simulink model "communicationExcavatorCANOldShit"  (R2025a)
settings: Solver=VariableStepAuto  StartTime=0.0  StopTime=Inf  RelTol=1e-3
undefined symbols (not defined in the file or in its folder): canChannel, SampleTime
libraries: canlib x10, canmsglib x8, simulink_extras x4, simulink x3, aerolibanimutils x1, sl3dlib x1
settings Model: Creator=Viktor Traktor  LastModifiedBy=Viktor Traktor
settings SolverCC: DecoupledContinuousIntegration=on

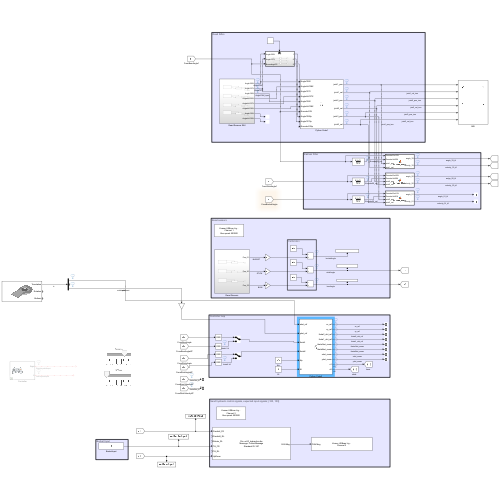
[thumbnail: Simulink's stored preview of the top-level diagram]
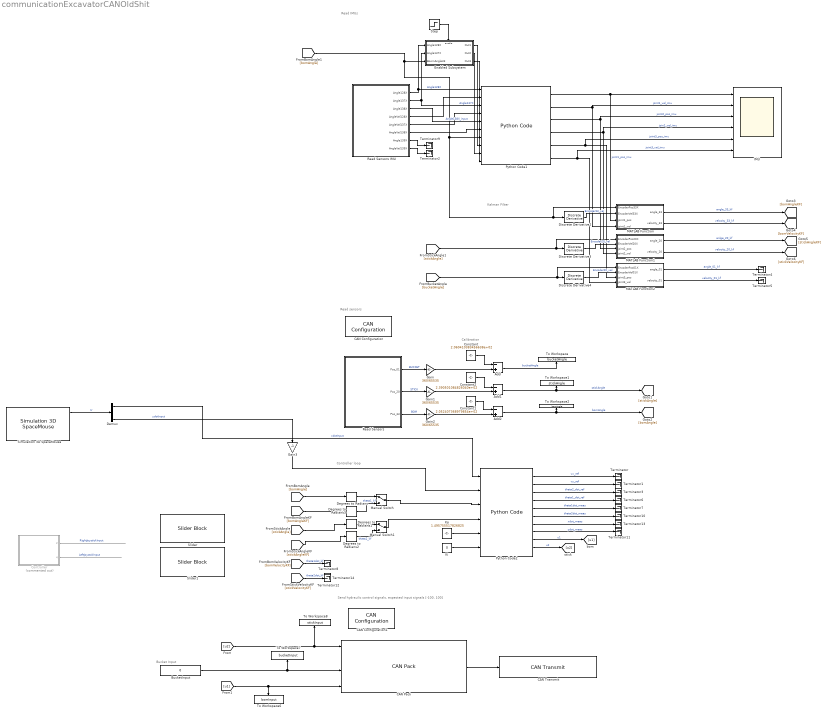
== system communicationExcavatorCANOldShit ==
  note: Controller loop
  note: Read sensors
  note: Send hydraulic control signals, expected input signals [-100, 100]
  note: Calibration
  note: Bucket Input
  note: Kalman Filter
  note: Read IMUs
  Add : Sum  Inputs=-+
  Add1 : Sum  Inputs=-+
  Add2 : Sum  Inputs=-+
  BucketInput : Constant  Value=0
  CAN Configuration : canlib/CAN Configuration  BlockHandle=6751.0004  Device=Kvaser USBcan Light 1 (Channel 1)  DeviceMenu=Kvaser USBcan Light 1 (Channel 1)  ObjConstructor=canChannel('Kvaser', 'USBcan Light 1', 1)  BusSpeed=500000  EnableBitParameters=off  SJW=1  TSEG1=4  TSEG2=3  NSamples=1  AckMode=Normal
  CAN Configuration1 : canlib/CAN Configuration  BlockHandle=6752.0004  Device=Kvaser USBcan Light 1 (Channel 2)  DeviceMenu=Kvaser USBcan Light 1 (Channel 2)  ObjConstructor=canChannel('Kvaser', 'USBcan Light 1', 2)  BusSpeed=500000  EnableBitParameters=off  SJW=1  TSEG1=4  TSEG2=3  NSamples=1  AckMode=Normal
  CAN Pack : canmsglib/CAN Pack  CANdbFile=C:\Users\Viktor Traktor\IQAN\ec20_hydraulics.dbc  MsgList=ControlMessage  MsgName=ControlMessage  MsgIDType=Standard (11-bit identifier)  MsgIdentifier=387  CANIDInput=off  MsgLength=6  Remote=off  ApplyMinMax=off  BusOutput=off  SignalInfo={'Parallell_FR','8','8','LE','signed','Standard','0','1','0','-Inf','Inf';'Parallelll_RL','0','8','LE','signed','Standard','0','1','0','-Inf','Inf';'Rotate_RL','40','8','LE','signed','Standard','0','1','0','-Inf','Inf';'Tilt_FR','24','8','LE','signed','Standard','0','1','0','-Inf','Inf';'Tilt_RL','32','8','LE','signed','Standard','0','1','0','-Inf','Inf';'UpDown','16','8','LE','signed','Standard','0','1','0','-Inf','Inf'}
      settings: LibrarySourceBlock=canlib/CAN Pack  DataFormat=CANdb specified signals
  CAN Transmit : canlib/CAN Transmit  BlockHandle=6761.0004  Device=Kvaser USBcan Light 1 (Channel 2)  DeviceMenu=Kvaser USBcan Light 1 (Channel 2)  ObjConstructor=canChannel('Kvaser', 'USBcan Light 1', 2)  EnableEventTransmit=off  EnablePeriodicTransmit=off  MessagePeriod=1.000
  Constant : Constant  Value=2.060410383456638e+02
  Constant1 : Constant  Value=2.052407368979854e+02
  Constant2 : Constant  Value=2.390501084826040e+02
  Controller : Subsystem  Commented=on
      mask Display: image('controller.png', [0,0,20,0,100,100]);
  Degrees to Radians{,1..3} (4 alike) : simulink_extras/Transformations/Degrees to Radians
  Demux : Demux  Outputs=3
  Discrete Derivative2 : simulink/Discrete/Discrete Derivative  gainval=1.0  ICPrevScaledInput=0.0  OutMin=[]  OutMax=[]  OutDataType=fixdt(1, 16)  OutScaling=2^-10  DoSatur=off
  Discrete Derivative3 : simulink/Discrete/Discrete Derivative  gainval=1.0  ICPrevScaledInput=0.0  OutMin=[]  OutMax=[]  OutDataType=fixdt(1, 16)  OutScaling=2^-10  DoSatur=off
  Discrete Derivative4 : simulink/Discrete/Discrete Derivative  gainval=1.0  ICPrevScaledInput=0.0  OutMin=[]  OutMax=[]  OutDataType=fixdt(1, 16)  OutScaling=2^-10  DoSatur=off
  Enabled Subsystem : Subsystem  TreatAsAtomicUnit=on
  Gain : Gain  Gain=360/65535
  Gain1 : Gain  Gain=360/65535
  Gain2 : Gain  Gain=360/65535
  Gain3 : Gain  Gain=-1
  IMU : Scope  NumInputPorts=6
      settings: ActiveDisplayYMinimum=240.03476604985391  ActiveDisplayYMaximum=241.62685406904103
  Ki : Constant  Value=0
  Kp : Constant  Value=1.495755517826825
  MATLAB Function : MATLAB Function  TreatAsAtomicUnit=on
  MATLAB Function1 : MATLAB Function  TreatAsAtomicUnit=on
  MATLAB Function2 : MATLAB Function  TreatAsAtomicUnit=on
  Manual Switch : ManualSwitch
  Manual Switch1 : ManualSwitch
  Python Code1 : PythonCode  OutputCode=|
      | # Computation
      | 
      | #print(Angle128X)
      | 
      | if Angle128X > 180:
      |     Angle128X = abs(Angle128X) - 360
      |     
      | if Angle137X < 20:
      |     Angle137X = abs(Angle137X)+360
      |     
      | if Angle138X > 270:
      |     Angle138X = abs(Angle138X) - 360
      |     
      | #print("///")
      | #print(Angle128X)
      | 
      | 
      | joint1_pos = Angle137X -270 + Angle128X - (Angle137Xp-270 + Angle128Xp - Encoder33Xp)
      | joint1_vel = -(AngleVel137X - AngleVel128X)
      | 
      | joint2_pos = 180 + (90 - joint1_pos) + Angle138X
      | joint2_vel = AngleVel138X - joint1_vel
      | 
      | joint3_pos = 0
      | joint3_vel = 0
  Python Code2 : PythonCode  OutputCode=|  SampleTime=SampleTime  max_joint_vel1=0.5  max_joint_vel2=0.5  SampleTime=0.01
      | import numpy as np
      | 
      | # Inputs:
      | #   xdot_ref, ydot_ref in [-1, 1]   (joystick commands, normalized)
      | #   theta1, theta2 [rad]            (joint angles)
      | #   max_joint_vel1, max_joint_vel2  [rad/s]
      | #
      | # Outputs:
      | #   u1, u2 in [-100, 100]           (valve commands)
      | 
      | 
      | # -------------------------------------------------------------------
      | # Constants
      | # -------------------------------------------------------------------
      | DT = 0.01  # time step [s]
      | 
      | VX_MAX = 0.5  # max Cartesian speed along x [m/s]
      | VY_MAX = 0.5  # max Cartesian speed along y [m/s]
      | 
      | AXIS_DEADZONE_NORM = 0.09   # joystick deadzone in normalized units [-1, 1]
      | 
      | M0 = 0.08      # shaping deadzone
      | P_SHAPE = 2.0  # shaping exponent
      | 
      | # Link lengths [m]
      | L1 = 1903.392e-3
      | L2 = 1351.485e-3
      | L3 = 590.267e-3  # not using the bucket angle here
      | 
      | # Joint-space PID gains
      | #Kp = .7
      | #Ki = 0.3
      | Kd = 0.0
      | 
      | # -------------------------------------------------------------------
      | # 1) Joystick -> Cartesian velocity reference (axis-locked)
      | # -------------------------------------------------------------------
      | 
      | # default (deadzone or no input)
      | vx_ref = 0.0
      | vy_ref = 0.0
      | 
      | if not (abs(xdot_ref) <= AXIS_DEADZONE_NORM and abs(ydot_ref) <= AXIS_DEADZONE_NORM):
      | 
      |     # Decide dominant axis: X-mode or Y-mode
      |     if abs(xdot_ref) > abs(ydot_ref):
      |         # X-mode
      |         vel_ref = xdot_ref
      |         v_max = VX_MAX
      | 
      |         if abs(vel_ref) > AXIS_DEADZONE_NORM:
      |             # sign
      |             sign = 1.0 if vel_ref >= 0.0 else -1.0
      |             # normalize magnitude into [0,1] after deadzone
      |             mag_norm = (abs(vel_ref) - AXIS_DEADZONE_NORM) / (1.0 - AXIS_DEADZONE_NORM)
      | 
      |             # shaping
      |             if mag_norm <= M0:
      |                 f = 0.0
      |             else:
      |                 r = (mag_norm - M0) / (1.0 - M0)
      |                 f = r ** P_SHAPE
      | 
      |             vx_ref = sign * v_max * f
      |             vy_ref = 0.0
      | 
      |     else:
      |         # Y-mode
      |         vel_ref = ydot_ref
      |         v_max = VY_MAX
      | 
      |         if abs(vel_ref) > AXIS_DEADZONE_NORM:
      |             sign = 1.0 if vel_ref >= 0.0 else -1.0
      |             mag_norm = (abs(vel_ref) - AXIS_DEADZONE_NORM) / (1.0 - AXIS_DEADZONE_NORM)
      | 
      |             if mag_norm <= M0:
      |                 f = 0.0
      |             else:
      |                 r = (mag_norm - M0) / (1.0 - M0)
      |                 f = r ** P_SHAPE
      | 
      |             vy_ref = sign * v_max * f
      |             vx_ref = 0.0
      | 
      | xydot_ref = np.array([vx_ref, vy_ref])
      | 
      | # -------------------------------------------------------------------
      | # 2) Jacobian and joint velocity reference (IK)
      | # -------------------------------------------------------------------
      | 
      | J11 = -L1 * np.sin(theta1) - L2 * np.sin(theta1 + theta2)
      | J12 = -L2 * np.sin(theta1 + theta2)
      | J21 =  L1 * np.cos(theta1) + L2 * np.cos(theta1 + theta2)
      | J22 =  L2 * np.cos(theta1 + theta2)
      | 
      | J = np.array([[J11, J12],
      |               [J21, J22]])
      | 
      | Jpinv = np.linalg.pinv(J)
      | 
      | theta_dot_ref_vec = Jpinv @ xydot_ref
      | theta1_dot_ref = float(theta_dot_ref_vec[0])
      | theta2_dot_ref = float(theta_dot_ref_vec[1])
      | 
      | theta1_dot_ref = float(np.clip(theta1_dot_ref, -max_joint_vel1, max_joint_vel1))
      | theta2_dot_ref = float(np.clip(theta2_dot_ref, -max_joint_vel2, max_joint_vel2))
      | theta_dot_ref_vec = np.array([theta1_dot_ref, theta2_dot_ref])
      | 
      | 
      | # -------------------------------------------------------------------
      | # 3) Measured joint velocities (finite difference)
      | # -------------------------------------------------------------------
      | 
      | if theta1_prev is None:
      |     theta1_prev = theta1
      | if theta2_prev is None:
      |     theta2_prev = theta2
      | 
      | theta1dot_meas = (theta1 - theta1_prev) / DT
      | theta2dot_meas = (theta2 - theta2_prev) / DT
      | 
      | theta1_prev = theta1
      | theta2_prev = theta2
      | 
      | thetadot_meas_vec = np.array([theta1dot_meas, theta2dot_meas])
      | 
      | 
      | # -------------------------------------------------------------------
      | # Logg detta i Simulink för: Cartesian measured velocity & error
      | # -------------------------------------------------------------------
      | 
      | xydot_meas = J @ thetadot_meas_vec
      | xdot_meas = float(xydot_meas[0])
      | ydot_meas = float(xydot_meas[1])
      | 
      | xydot_error = xydot_ref - xydot_meas
      | xdot_error = float(xydot_error[0])
      | ydot_error = float(xydot_error[1])
      | 
      | 
      | # -------------------------------------------------------------------
      | # 4) Joint velocity error (for joint-space PID)
      | # -------------------------------------------------------------------
      | 
      | thetadot_error = theta_dot_ref_vec - thetadot_meas_vec
      | theta1dot_error = float(thetadot_error[0])
      | theta2dot_error = float(thetadot_error[1])
      | 
      | 
      | # -------------------------------------------------------------------
      | # 5) Integral term (trapezoidal)
      | # -------------------------------------------------------------------
      | 
      | if thetadot1_error_prev is None:
      |     thetadot1_error_prev = 0.0
      | if thetadot2_error_prev is None:
      |     thetadot2_error_prev = 0.0
      | 
      | theta1dot_error_integral = (
      |     (theta1dot_error + thetadot1_error_prev) * DT / 2.0
      |     + thetadot1_error_integral_prev
      | )
      | theta2dot_error_integral = (
      |     (theta2dot_error + thetadot2_error_prev) * DT / 2.0
      |     + thetadot2_error_integral_prev
      | )
      | 
      | thetadot1_error_integral_prev = theta1dot_error_integral
      | thetadot2_error_integral_prev = theta2dot_error_integral
      | 
      | thetadot_error_integral = np.array([
      |     theta1dot_error_integral,
      |     theta2dot_error_integral
      | ])
      | 
      | 
      | # -------------------------------------------------------------------
      | # 6) Derivative term
      | # -------------------------------------------------------------------
      | 
      | theta1dot_error_derivative = (theta1dot_error - thetadot1_error_prev) / DT
      | theta2dot_error_derivative = (theta2dot_error - thetadot2_error_prev) / DT
      | 
      | thetadot_error_derivative = np.array([
      |     theta1dot_error_derivative,
      |     theta2dot_error_derivative
      | ])
      | 
      | thetadot1_error_prev = theta1dot_error
      | thetadot2_error_prev = theta2dot_error
      | 
      | 
      | # -------------------------------------------------------------------
      | # 7) Joint-space PID to normalized valve control [-1, 1]
      | # -------------------------------------------------------------------
      | 
      | valve_control_norm_vec = Kp*thetadot_error + Ki*thetadot_error_integral + Kd*thetadot_error_derivative
      | 
      | valve_control_norm_vec = np.clip(valve_control_norm_vec, -1.0, 1.0)
      | 
      | control_1_norm = -float(valve_control_norm_vec[0])
      | control_2_norm = float(valve_control_norm_vec[1])
      | 
      | 
      | # -------------------------------------------------------------------
      | # 8) Scale normalized control to valve hardware range [-100, 100]
      | # -------------------------------------------------------------------
      | u1 = float(np.clip(control_1_norm * 100.0, -100.0, 100.0))
      | u2 = float(np.clip(control_2_norm * 100.0, -100.0, 100.0))
  Read Sensors : Subsystem
  Read Sensors IMU : Subsystem
  Simulation 3D SpaceMouse : sl3dlib/Simulation 3D/Hardware Interface/Simulation 3D SpaceMouse  Port=USB1  OutputType=Speed  Dominant=off  DisableTranslation=off  DisableRotation=off  NormalizeAngle=off  EnableLimit=off  PositionSensitivity=0.00058  RotationSensitivity=0.00001  InitialPosition=[0 0 0]  InitialRotation=[0 0 1 0]  PositionLow=[-100 -100 -100]  PositionUp=[100 100 100]
  Slider : SliderBlock  ScaleMax=2
  Slider1 : SliderBlock  ScaleMax=1
  Step : Step  Time=0.001  Before=1  After=0  SampleTime=0
  Terminator{,1..14} (15 alike) : Terminator
  To Workspace : ToWorkspace  VariableName=bucketAngle  SaveFormat=Timeseries  SampleTime=-1
  To Workspace1 : ToWorkspace  VariableName=stickAngle  SaveFormat=Timeseries  SampleTime=-1
  To Workspace2 : ToWorkspace  VariableName=bomAngle  SaveFormat=Timeseries  SampleTime=-1
  To Workspace6 : ToWorkspace  VariableName=bomInput  SaveFormat=Timeseries  SampleTime=-1
  To Workspace7 : ToWorkspace  VariableName=bucketInput  SaveFormat=Timeseries  SampleTime=-1
  To Workspace8 : ToWorkspace  VariableName=stickInput  SaveFormat=Timeseries  SampleTime=-1
  wires:
  CAN Pack/1 -> CAN Transmit/1
  Add/1 -> To Workspace/1  "bucketAngle"
  Read Sensors/3(Pos_33) -> Gain2/1  "BOM"
  Add2/1 -> [bomAngle], To Workspace2/1  "bomAngle"
  Gain1/1 -> Add1/2
  Constant/1 -> Add/1
  Add1/1 -> [stickAngle], To Workspace1/1  "stickAngle"
  Gain/1 -> Add/2
  Constant1/1 -> Add2/1
  Constant2/1 -> Add1/1
  Read Sensors/1(Pos_01) -> Gain/1  "BUCKET"
  Read Sensors/2(Pos_20) -> Gain1/1  "STICK"
  Gain2/1 -> Add2/2
  BucketInput/1 -> CAN Pack/4, To Workspace7/1
  [u2] -> CAN Pack/1, To Workspace8/1
  [u1] -> CAN Pack/6, To Workspace6/1
  [stickAngle] -> Degrees to Radians1/1
  Python Code2/3 -> Terminator3/1  "theta2_dot_ref"
  Python Code2/7 -> Terminator13/1  "xdot_meas"
  Python Code2/5 -> Terminator7/1  "theta1dot_meas"
  Python Code2/10 -> [u2]  "u2"
  Python Code2/4 -> Terminator6/1  "theta1_dot_ref"
  Python Code2/6 -> Terminator10/1  "theta2dot_meas"
  Controller/1(2) -> ?  "RightJoystickInput"
  Python Code2/2 -> Terminator1/1  "vy_ref"
  Controller/2(4) -> ?  "LeftJoystckInput"
  Python Code2/9 -> [u1]  "u1"
  Python Code2/8 -> Terminator11/1  "ydot_meas"
  Python Code2/1 -> Terminator/1  "vx_ref"
  Kp/1 -> Python Code2/5
  Ki/1 -> Python Code2/6
  Demux/1 -> Python Code2/1  "xdotInput"
  Demux/3 -> Gain3/1  "ydotInput"
  Gain3/1 -> Python Code2/2
  Simulation 3D SpaceMouse/1 -> Demux/1  "tr"
  MATLAB Function2/1(angle_01) -> Terminator4/1  "angle_01_kf"
  Python Code1/6 -> IMU/6, MATLAB Function2/4(joint3_vel)  "joint3_vel_imu"
  Read Sensors IMU/5(AngleVel137X) -> Python Code1/4
  Read Sensors IMU/4(AngleVel128X) -> Python Code1/2
  Read Sensors IMU/8(AngleVel139X) -> Terminator2/1
  Discrete Derivative3/1 -> MATLAB Function1/2(EncoderVel20X)  "Encoder20_vel"
  Read Sensors IMU/2(Angle137X) -> Python Code1/3, Enabled Subsystem/2(Angle137X)  "Angle137X"
  MATLAB Function/2(velocity_33) -> [bomVelocityKF]  "velocity_33_kf"
  Enabled Subsystem/2(Out2) -> Python Code1/9
  [stickAngle] -> MATLAB Function1/1(EncoderPos20X), Discrete Derivative3/1
  Python Code1/5 -> IMU/5, MATLAB Function2/3(joint3_pos)  "joint3_pos_imu"
  Read Sensors IMU/7(Angle139X) -> Terminator9/1
  Python Code1/3 -> IMU/3, MATLAB Function1/3(joint2_pos)  "joint2_pos_imu"
  Discrete Derivative2/1 -> MATLAB Function/2(EncoderVel33X)  "Encoder33_vel"
  Step/1 -> Enabled Subsystem/Enable
  Enabled Subsystem/3(Out3) -> Python Code1/10
  [bucketAngle] -> MATLAB Function2/1(EncoderPos01X), Discrete Derivative4/1
  Read Sensors IMU/1(Angle128X) -> Python Code1/1, Enabled Subsystem/1(Angle128X)  "Angle128X"
  Enabled Subsystem/1(Out1) -> Python Code1/8
  Discrete Derivative4/1 -> MATLAB Function2/2(EncoderVel01X)  "Encoder20_vel"
  Python Code1/2 -> IMU/2, MATLAB Function/4(joint1_vel)  "joint1_vel_imu"
  Read Sensors IMU/3(Angle138X) -> Python Code1/5  "Angle138X_input"
  Read Sensors IMU/6(AngleVel138X) -> Python Code1/6
  MATLAB Function/1(angle_33) -> [bomAngleKF]  "angle_33_kf"
  Python Code1/1 -> MATLAB Function/3(joint1_pos), IMU/1  "joint1_pos_imu"
  MATLAB Function2/2(velocity_01) -> Terminator5/1  "velocity_01_kf"
  MATLAB Function1/2(velocity_20) -> [stickVelocityKF]  "velocity_20_kf"
  MATLAB Function1/1(angle_20) -> [stickAngleKF]  "anlge_20_kf"
  Python Code1/4 -> IMU/4, MATLAB Function1/4(joint2_vel)  "join2_vel_imu"
  [bomAngle] -> MATLAB Function/1(EncoderPos33X), Discrete Derivative2/1, Python Code1/7, Enabled Subsystem/3(BoomAngle33)
  [bomAngle] -> Degrees to Radians/1
  Degrees to Radians/1 -> Manual Switch/1
  Manual Switch/1 -> Python Code2/3
  Manual Switch1/1 -> Python Code2/4
  Degrees to Radians1/1 -> Manual Switch1/1
  [stickAngleKF] -> Degrees to Radians2/1
  Degrees to Radians2/1 -> Manual Switch1/2  "theta2_kf"
  Degrees to Radians3/1 -> Manual Switch/2  "theta1_kf"
  [bomAngleKF] -> Degrees to Radians3/1
  [bomVelocityKF] -> Terminator8/1  "theta1dot_kf"
  [stickVelocityKF] -> Terminator14/1  "theta2dot_kf"

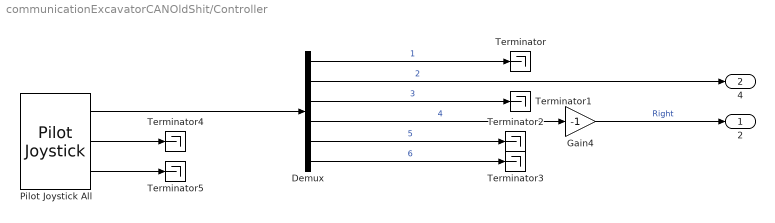
== system communicationExcavatorCANOldShit/Controller ==
  Demux : Demux  Outputs=6
  Gain4 : Gain  Gain=-1
  Pilot Joystick All : aerolibanimutils/Pilot Joystick  JoystickID=Joystick2  OutputConfiguration=AllOutputs  SampleTime=1/50
      settings: LibrarySourceBlock=aerolibanimutils/Pilot Joystick All
  Terminator{,1..5} (6 alike) : Terminator
  2 : Outport
  4 : Outport  Port=2
  wires:
  Demux/6 -> Terminator3/1  "6"
  Demux/5 -> Terminator2/1  "5"
  Pilot Joystick All/3 -> Terminator5/1
  Pilot Joystick All/1 -> Demux/1
  Demux/1 -> Terminator/1  "1"
  Demux/4 -> Gain4/1  "4"
  Pilot Joystick All/2 -> Terminator4/1
  Demux/3 -> Terminator1/1  "3"
  Demux/2 -> 4/1  "2"
  Gain4/1 -> 2/1  "Right"

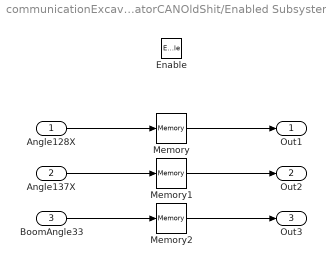
== system communicationExcavatorCANOldShit/Enabled Subsystem ==
  Angle128X : Inport
  Angle137X : Inport  Port=2
  BoomAngle33 : Inport  Port=3
  Enable : EnablePort
  Memory : Memory
  Memory1 : Memory
  Memory2 : Memory
  Out1 : Outport
  Out2 : Outport  Port=2
  Out3 : Outport  Port=3
  wires:
  Angle128X/1 -> Memory/1
  Memory/1 -> Out1/1
  Angle137X/1 -> Memory1/1
  BoomAngle33/1 -> Memory2/1
  Memory1/1 -> Out2/1
  Memory2/1 -> Out3/1

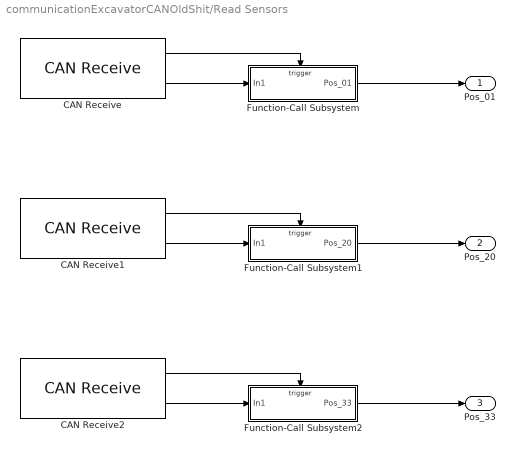
== system communicationExcavatorCANOldShit/Read Sensors ==
  CAN Receive : canlib/CAN Receive  BlockHandle=6913.0005  Device=Kvaser USBcan Light 1 (Channel 1)  DeviceMenu=Kvaser USBcan Light 1 (Channel 1)  ObjConstructor=canChannel('Kvaser', 'USBcan Light 1', 1)  EnableStandardIDsFilter=off  StdIDsCombo=Allow all  StandardIDs=0  EnableExtendedIDsFilter=off  ExtIDsCombo=Allow all  ExtendedIDs=0  SampleTime=0.01  MsgsPerTimestep=all  InternalFilterUpdateStatus=on  BusOutput=off
  CAN Receive1 : canlib/CAN Receive  BlockHandle=6917.0005  Device=Kvaser USBcan Light 1 (Channel 1)  DeviceMenu=Kvaser USBcan Light 1 (Channel 1)  ObjConstructor=canChannel('Kvaser', 'USBcan Light 1', 1)  EnableStandardIDsFilter=off  StdIDsCombo=Allow all  StandardIDs=0  EnableExtendedIDsFilter=off  ExtIDsCombo=Allow all  ExtendedIDs=0  SampleTime=0.01  MsgsPerTimestep=all  InternalFilterUpdateStatus=on  BusOutput=off
  CAN Receive2 : canlib/CAN Receive  BlockHandle=6920.0002  Device=Kvaser USBcan Light 1 (Channel 1)  DeviceMenu=Kvaser USBcan Light 1 (Channel 1)  ObjConstructor=canChannel('Kvaser', 'USBcan Light 1', 1)  EnableStandardIDsFilter=off  StdIDsCombo=Allow all  StandardIDs=0  EnableExtendedIDsFilter=off  ExtIDsCombo=Allow all  ExtendedIDs=0  SampleTime=0.01  MsgsPerTimestep=all  InternalFilterUpdateStatus=on  BusOutput=off
  Function-Call Subsystem : Subsystem  TreatAsAtomicUnit=on
  Function-Call Subsystem1 : Subsystem  TreatAsAtomicUnit=on
  Function-Call Subsystem2 : Subsystem  TreatAsAtomicUnit=on
  Pos_01 : Outport
  Pos_20 : Outport  Port=2
  Pos_33 : Outport  Port=3
  wires:
  CAN Receive/2 -> Function-Call Subsystem/1(In1)
  CAN Receive1/2 -> Function-Call Subsystem1/1(In1)
  CAN Receive/1 -> Function-Call Subsystem/Trigger
  CAN Receive2/2 -> Function-Call Subsystem2/1(In1)
  Function-Call Subsystem2/1(Pos_33) -> Pos_33/1
  Function-Call Subsystem/1(Pos_01) -> Pos_01/1
  CAN Receive2/1 -> Function-Call Subsystem2/Trigger
  CAN Receive1/1 -> Function-Call Subsystem1/Trigger
  Function-Call Subsystem1/1(Pos_20) -> Pos_20/1

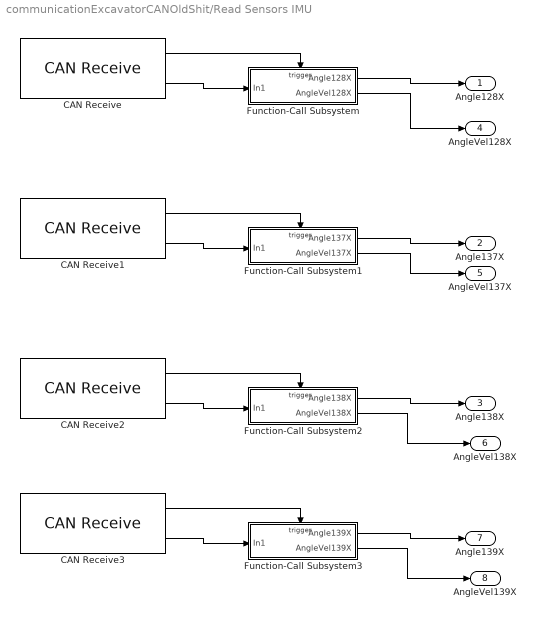
== system communicationExcavatorCANOldShit/Read Sensors IMU ==
  CAN Receive : canlib/CAN Receive  BlockHandle=8637.0006  Device=Kvaser USBcan Light 1 (Channel 1)  DeviceMenu=Kvaser USBcan Light 1 (Channel 1)  ObjConstructor=canChannel('Kvaser', 'USBcan Light 1', 1)  EnableStandardIDsFilter=off  StdIDsCombo=Allow all  StandardIDs=0  EnableExtendedIDsFilter=off  ExtIDsCombo=Allow all  ExtendedIDs=0  SampleTime=0.01  MsgsPerTimestep=all  InternalFilterUpdateStatus=on  BusOutput=off
  CAN Receive1 : canlib/CAN Receive  BlockHandle=8640.0006  Device=Kvaser USBcan Light 1 (Channel 1)  DeviceMenu=Kvaser USBcan Light 1 (Channel 1)  ObjConstructor=canChannel('Kvaser', 'USBcan Light 1', 1)  EnableStandardIDsFilter=off  StdIDsCombo=Allow all  StandardIDs=0  EnableExtendedIDsFilter=off  ExtIDsCombo=Allow all  ExtendedIDs=0  SampleTime=0.01  MsgsPerTimestep=all  InternalFilterUpdateStatus=on  BusOutput=off
  CAN Receive2 : canlib/CAN Receive  BlockHandle=8643.0006  Device=Kvaser USBcan Light 1 (Channel 1)  DeviceMenu=Kvaser USBcan Light 1 (Channel 1)  ObjConstructor=canChannel('Kvaser', 'USBcan Light 1', 1)  EnableStandardIDsFilter=off  StdIDsCombo=Allow all  StandardIDs=0  EnableExtendedIDsFilter=off  ExtIDsCombo=Allow all  ExtendedIDs=0  SampleTime=0.01  MsgsPerTimestep=all  InternalFilterUpdateStatus=on  BusOutput=off
  CAN Receive3 : canlib/CAN Receive  BlockHandle=8646.0005  Device=Kvaser USBcan Light 1 (Channel 1)  DeviceMenu=Kvaser USBcan Light 1 (Channel 1)  ObjConstructor=canChannel('Kvaser', 'USBcan Light 1', 1)  EnableStandardIDsFilter=off  StdIDsCombo=Allow all  StandardIDs=0  EnableExtendedIDsFilter=off  ExtIDsCombo=Allow all  ExtendedIDs=0  SampleTime=0.01  MsgsPerTimestep=all  InternalFilterUpdateStatus=on  BusOutput=off
  Function-Call Subsystem : Subsystem  TreatAsAtomicUnit=on
  Function-Call Subsystem1 : Subsystem  TreatAsAtomicUnit=on
  Function-Call Subsystem2 : Subsystem  TreatAsAtomicUnit=on
  Function-Call Subsystem3 : Subsystem  TreatAsAtomicUnit=on
  Angle128X : Outport
  Angle137X : Outport  Port=2
  Angle138X : Outport  Port=3
  AngleVel128X : Outport  Port=4
  AngleVel137X : Outport  Port=5
  AngleVel138X : Outport  Port=6
  Angle139X : Outport  Port=7
  AngleVel139X : Outport  Port=8
  wires:
  Function-Call Subsystem1/1(Angle137X) -> Angle137X/1
  CAN Receive1/1 -> Function-Call Subsystem1/Trigger
  CAN Receive2/1 -> Function-Call Subsystem2/Trigger
  Function-Call Subsystem/1(Angle128X) -> Angle128X/1
  Function-Call Subsystem2/1(Angle138X) -> Angle138X/1
  CAN Receive2/2 -> Function-Call Subsystem2/1(In1)
  CAN Receive/1 -> Function-Call Subsystem/Trigger
  CAN Receive1/2 -> Function-Call Subsystem1/1(In1)
  CAN Receive/2 -> Function-Call Subsystem/1(In1)
  Function-Call Subsystem/2(AngleVel128X) -> AngleVel128X/1
  Function-Call Subsystem1/2(AngleVel137X) -> AngleVel137X/1
  Function-Call Subsystem2/2(AngleVel138X) -> AngleVel138X/1
  Function-Call Subsystem3/2(AngleVel139X) -> AngleVel139X/1
  CAN Receive3/2 -> Function-Call Subsystem3/1(In1)
  Function-Call Subsystem3/1(Angle139X) -> Angle139X/1
  CAN Receive3/1 -> Function-Call Subsystem3/Trigger

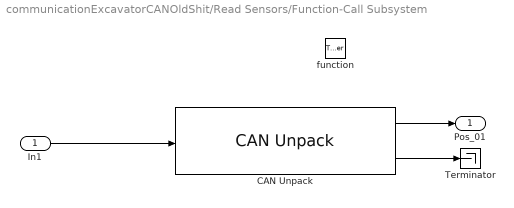
== system communicationExcavatorCANOldShit/Read Sensors/Function-Call Subsystem ==
  In1 : Inport
  function : TriggerPort  TriggerType=function-call  VariantControl=(inherit)
  CAN Unpack : canmsglib/CAN Unpack  CANdbFile=C:\Users\Viktor Traktor\Downloads\VolvoExcavator\systemIdentificationVolvo\ec20_kth.dbc  MsgList=Rot_01  MsgName=Rot_01  MsgIDType=Extended (29-bit identifier)  MsgIdentifier=419408385  MsgLength=8  SignalInfo={'SnsrPos_01','0','32','LE','unsigned','Standard','0','1','0','0','4294967295';'SnsrRPM_01','32','16','LE','unsigned','Standard','0','1','0','0','65535'}  IDPort=off  TimestampPort=off  ErrorPort=off  RemotePort=off  LengthPort=off  StatusPort=off  ApplyMinMax=off
      settings: LibrarySourceBlock=canlib/CAN Unpack  DataFormat=CANdb specified signals
  Terminator : Terminator
  Pos_01 : Outport
  wires:
  In1/1 -> CAN Unpack/1
  CAN Unpack/1 -> Pos_01/1
  CAN Unpack/2 -> Terminator/1

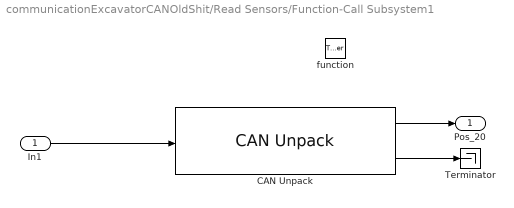
== system communicationExcavatorCANOldShit/Read Sensors/Function-Call Subsystem1 ==
  In1 : Inport
  function : TriggerPort  TriggerType=function-call  VariantControl=(inherit)
  CAN Unpack : canmsglib/CAN Unpack  CANdbFile=C:\Users\Viktor Traktor\Downloads\VolvoExcavator\systemIdentificationVolvo\ec20_kth.dbc  MsgList=Rot_20  MsgName=Rot_20  MsgIDType=Extended (29-bit identifier)  MsgIdentifier=419408416  MsgLength=8  SignalInfo={'SnsrPos_20','0','32','LE','unsigned','Standard','0','1','0','0','4294967295';'SnsrRPM_20','32','16','LE','unsigned','Standard','0','1','0','0','65535'}  IDPort=off  TimestampPort=off  ErrorPort=off  RemotePort=off  LengthPort=off  StatusPort=off  ApplyMinMax=off
      settings: LibrarySourceBlock=canlib/CAN Unpack  DataFormat=CANdb specified signals
  Terminator : Terminator
  Pos_20 : Outport
  wires:
  CAN Unpack/1 -> Pos_20/1
  In1/1 -> CAN Unpack/1
  CAN Unpack/2 -> Terminator/1

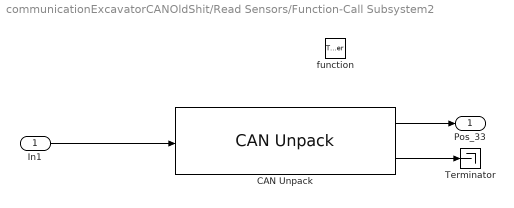
== system communicationExcavatorCANOldShit/Read Sensors/Function-Call Subsystem2 ==
  In1 : Inport
  function : TriggerPort  TriggerType=function-call  VariantControl=(inherit)
  CAN Unpack : canmsglib/CAN Unpack  CANdbFile=C:\Users\Viktor Traktor\Downloads\VolvoExcavator\systemIdentificationVolvo\ec20_kth.dbc  MsgList=Rot_33  MsgName=Rot_33  MsgIDType=Extended (29-bit identifier)  MsgIdentifier=419408435  MsgLength=8  SignalInfo={'SnsrPos_33','0','32','LE','unsigned','Standard','0','1','0','0','4294967295';'SnsrRPM_33','32','16','LE','unsigned','Standard','0','1','0','0','65535'}  IDPort=off  TimestampPort=off  ErrorPort=off  RemotePort=off  LengthPort=off  StatusPort=off  ApplyMinMax=off
      settings: LibrarySourceBlock=canlib/CAN Unpack  DataFormat=CANdb specified signals
  Terminator : Terminator
  Pos_33 : Outport
  wires:
  In1/1 -> CAN Unpack/1
  CAN Unpack/1 -> Pos_33/1
  CAN Unpack/2 -> Terminator/1

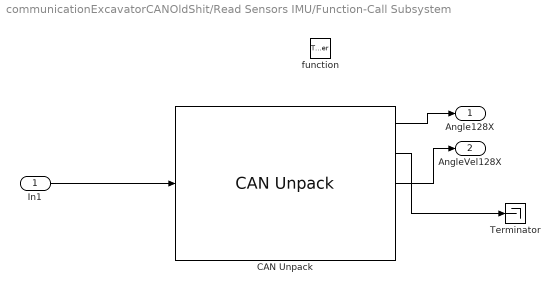
== system communicationExcavatorCANOldShit/Read Sensors IMU/Function-Call Subsystem ==
  In1 : Inport
  function : TriggerPort  TriggerType=function-call  VariantControl=(inherit)
  CAN Unpack : canmsglib/CAN Unpack  CANdbFile=C:\Users\Viktor Traktor\Downloads\VolvoExcavator\systemIdentificationVolvo\ec20_kth.dbc  MsgList=IMU_XAxis_128  MsgName=IMU_XAxis_128  MsgIDType=Extended (29-bit identifier)  MsgIdentifier=251592832  MsgLength=8  SignalInfo={'AngleXAxis_128','0','16','LE','unsigned','Standard','0','0.007813','0','0','512.025';'AngularAccelerationXAxis_128','32','16','LE','unsigned','Standard','0','0.03125','-1000','-1000','1047.9688';'AngularVelocityXAxis_128','16','16','LE','unsigned','Standard','0','0.007813','-250','-250','262.025';'CRC_Xaxis_128','56','8','LE','unsigned','Standard','0','1','0','0','255';'Counter_Xaxis_128','48','8','LE','unsigned','Standard','0','1','0','0','255'}  IDPort=off  TimestampPort=off  ErrorPort=off  RemotePort=off  LengthPort=off  StatusPort=off  ApplyMinMax=off
      settings: LibrarySourceBlock=canlib/CAN Unpack  DataFormat=CANdb specified signals
  Terminator : Terminator
  Angle128X : Outport
  AngleVel128X : Outport  Port=2
  wires:
  CAN Unpack/2 -> Terminator/1
  CAN Unpack/1 -> Angle128X/1
  In1/1 -> CAN Unpack/1
  CAN Unpack/3 -> AngleVel128X/1

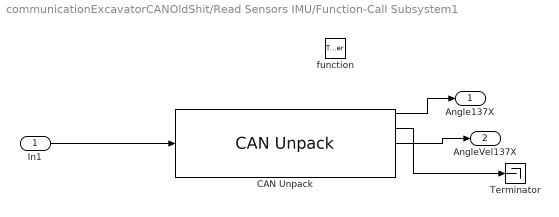
== system communicationExcavatorCANOldShit/Read Sensors IMU/Function-Call Subsystem1 ==
  In1 : Inport
  function : TriggerPort  TriggerType=function-call  VariantControl=(inherit)
  CAN Unpack : canmsglib/CAN Unpack  CANdbFile=C:\Users\Viktor Traktor\Downloads\VolvoExcavator\systemIdentificationVolvo\ec20_kth.dbc  MsgList=IMU_XAxis_137  MsgName=IMU_XAxis_137  MsgIDType=Extended (29-bit identifier)  MsgIdentifier=251592841  MsgLength=8  SignalInfo={'AngleXAxis_137','0','16','LE','unsigned','Standard','0','0.007813','0','0','512.025';'AngularAccelerationXAxis_137','32','16','LE','unsigned','Standard','0','0.03125','-1000','-1000','1047.9688';'AngularVelocityXAxis_137','16','16','LE','unsigned','Standard','0','0.007813','-250','-250','262.025';'CRC_Xaxis_137','56','8','LE','unsigned','Standard','0','1','0','0','255';'Counter_Xaxis_137','48','8','LE','unsigned','Standard','0','1','0','0','255'}  IDPort=off  TimestampPort=off  ErrorPort=off  RemotePort=off  LengthPort=off  StatusPort=off  ApplyMinMax=off
      settings: LibrarySourceBlock=canlib/CAN Unpack  DataFormat=CANdb specified signals
  Terminator : Terminator
  Angle137X : Outport
  AngleVel137X : Outport  Port=2
  wires:
  CAN Unpack/2 -> Terminator/1
  In1/1 -> CAN Unpack/1
  CAN Unpack/1 -> Angle137X/1
  CAN Unpack/3 -> AngleVel137X/1

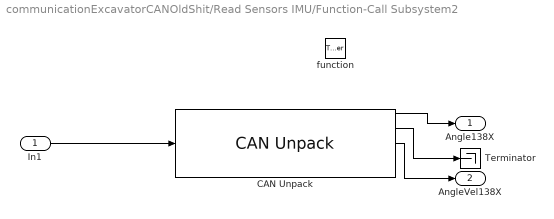
== system communicationExcavatorCANOldShit/Read Sensors IMU/Function-Call Subsystem2 ==
  In1 : Inport
  function : TriggerPort  TriggerType=function-call  VariantControl=(inherit)
  CAN Unpack : canmsglib/CAN Unpack  CANdbFile=C:\Users\Viktor Traktor\Downloads\VolvoExcavator\systemIdentificationVolvo\ec20_kth.dbc  MsgList=IMU_XAxis_138  MsgName=IMU_XAxis_138  MsgIDType=Extended (29-bit identifier)  MsgIdentifier=251592842  MsgLength=8  SignalInfo={'AngleXAxis_138','0','16','LE','unsigned','Standard','0','0.007813','0','0','512.025';'AngularAccelerationXAxis_138','32','16','LE','unsigned','Standard','0','0.03125','-1000','-1000','1047.9688';'AngularVelocityXAxis_138','16','16','LE','unsigned','Standard','0','0.007813','-250','-250','262.025';'CRC_Xaxis_138','56','8','LE','unsigned','Standard','0','1','0','0','255';'Counter_Xaxis_138','48','8','LE','unsigned','Standard','0','1','0','0','255'}  IDPort=off  TimestampPort=off  ErrorPort=off  RemotePort=off  LengthPort=off  StatusPort=off  ApplyMinMax=off
      settings: LibrarySourceBlock=canlib/CAN Unpack  DataFormat=CANdb specified signals
  Terminator : Terminator
  Angle138X : Outport
  AngleVel138X : Outport  Port=2
  wires:
  CAN Unpack/2 -> Terminator/1
  CAN Unpack/1 -> Angle138X/1
  In1/1 -> CAN Unpack/1
  CAN Unpack/3 -> AngleVel138X/1

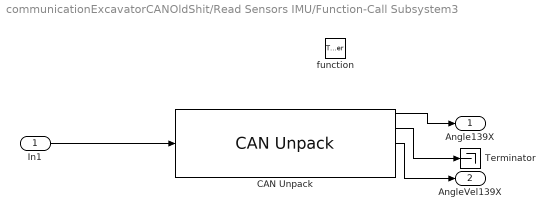
== system communicationExcavatorCANOldShit/Read Sensors IMU/Function-Call Subsystem3 ==
  In1 : Inport
  function : TriggerPort  TriggerType=function-call  VariantControl=(inherit)
  CAN Unpack : canmsglib/CAN Unpack  CANdbFile=C:\Users\Viktor Traktor\Downloads\VolvoExcavator\systemIdentificationVolvo\ec20_kth.dbc  MsgList=IMU_XAxis_139  MsgName=IMU_XAxis_139  MsgIDType=Extended (29-bit identifier)  MsgIdentifier=251592843  MsgLength=8  SignalInfo={'AngleXAxis_139','0','16','LE','unsigned','Standard','0','0.007813','0','0','512.025';'AngularAccelerationXAxis_139','32','16','LE','unsigned','Standard','0','0.03125','-1000','-1000','1047.9688';'AngularVelocityXAxis_139','16','16','LE','unsigned','Standard','0','0.007813','-250','-250','262.025';'CRC_Xaxis_139','56','8','LE','unsigned','Standard','0','1','0','0','255';'Counter_Xaxis_139','48','8','LE','unsigned','Standard','0','1','0','0','255'}  IDPort=off  TimestampPort=off  ErrorPort=off  RemotePort=off  LengthPort=off  StatusPort=off  ApplyMinMax=off
      settings: LibrarySourceBlock=canlib/CAN Unpack  DataFormat=CANdb specified signals
  Terminator : Terminator
  Angle139X : Outport
  AngleVel139X : Outport  Port=2
  wires:
  CAN Unpack/3 -> AngleVel139X/1
  In1/1 -> CAN Unpack/1
  CAN Unpack/1 -> Angle139X/1
  CAN Unpack/2 -> Terminator/1

== matlab function communicationExcavatorCANOldShit/MATLAB Function1 ==
  data: EncoderPos20X input; angle_20 output; EncoderVel20X input; joint2_pos input; joint2_vel input; velocity_20 output
function [angle_20, velocity_20]= kalman_block(EncoderPos20X, EncoderVel20X, joint2_pos, joint2_vel)
    persistent kf_20
    if isempty(kf_20)
        kf_20 = KalmanFilter(0.01);
    end
    
    kf_20.predict();
    kf_20.update(EncoderPos20X, EncoderVel20X, joint2_pos, joint2_vel);
    
    angle_20 = kf_20.x(1);
    velocity_20 = kf_20.x(2);

end

== matlab function communicationExcavatorCANOldShit/MATLAB Function ==
  data: EncoderPos33X input; angle_33 output; EncoderVel33X input; joint1_pos input; joint1_vel input; velocity_33 output
function [angle_33, velocity_33]= kalman_block(EncoderPos33X, EncoderVel33X, joint1_pos, joint1_vel)
    persistent kf_33
    if isempty(kf_33)
        kf_33 = KalmanFilter(0.01);
    end

    kf_33.predict();
    kf_33.update(EncoderPos33X, EncoderVel33X, joint1_pos, joint1_vel);
    
    angle_33 = kf_33.x(1);
    velocity_33 = kf_33.x(2);

end

== matlab function communicationExcavatorCANOldShit/MATLAB Function2 ==
  data: EncoderPos01X input; angle_01 output; EncoderVel01X input; joint3_pos input; joint3_vel input; velocity_01 output
function [angle_01, velocity_01]= kalman_block(EncoderPos01X, EncoderVel01X, joint3_pos, joint3_vel)
    persistent kf_01
    if isempty(kf_01)
        kf_01 = KalmanFilter(0.01);
    end
    
    kf_01.predict();
    kf_01.update(EncoderPos01X, EncoderVel01X, joint3_pos, joint3_vel);
    
    angle_01 = kf_01.x(1);
    velocity_01 = kf_01.x(2);

end
